simulink model "Quat"  (R2013b)
settings: Solver=ode45  StartTime=0.0  StopTime=100  RelTol=1e-3
undefined symbols (not defined in the file): IMU_DT, MagMeasure, P_init, Q, Rmag, wb, x_init
libraries: simulink x1
settings Model: Creator=Walker  LastModifiedBy=Walker

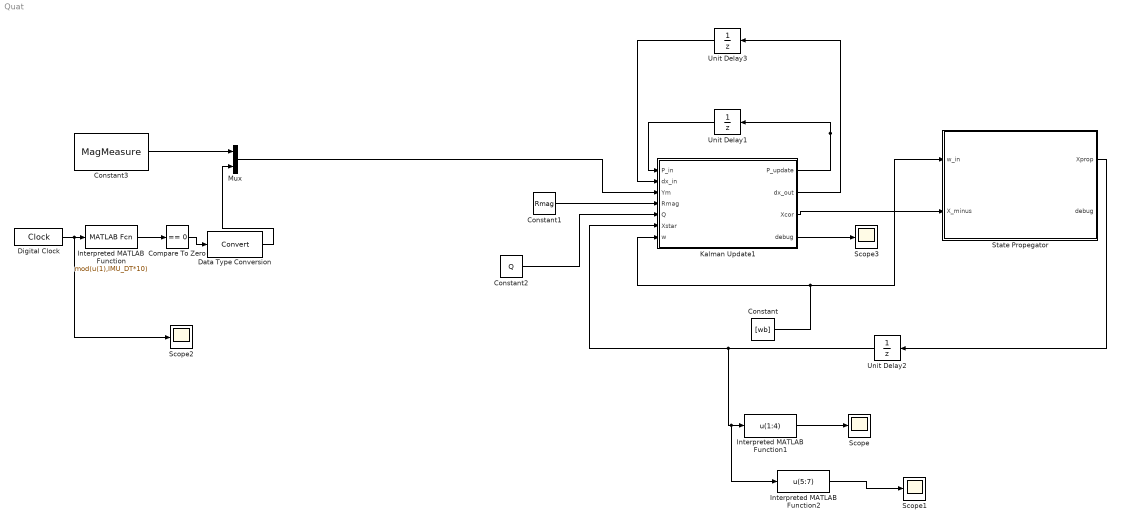
== system Quat ==
  Compare To Zero : simulink/Logic and Bit Operations/Compare To Zero  relop===  OutDataTypeStr=uint8
  Constant : Constant  Value=[wb]
  Constant1 : Constant  Value=Rmag
  Constant2 : Constant  Value=Q
  Constant3 : Constant  Value=MagMeasure
  Data Type Conversion : DataTypeConversion
  Digital Clock : DigitalClock  SampleTime=IMU_DT
  Interpreted MATLAB Function : MATLABFcn  MATLABFcn=mod(u(1),IMU_DT*10)
  Interpreted MATLAB Function1 : MATLABFcn  MATLABFcn=u(1:4)
  Interpreted MATLAB Function2 : MATLABFcn  MATLABFcn=u(5:7)
  Kalman Update1 : MATLAB Function  TreatAsAtomicUnit=on
  Mux : Mux  Inputs=2
  Scope{,1..3} (4 alike) : Scope
      Scope settings: TimeRange=10  YMin=-0.05  YMax=1
      Scope1 settings: YMin=-0.00325  YMax=0.00225
      Scope2 settings: YMin=10  YMax=130  SaveName=ScopeData2
      Scope3 settings: TimeRange=10  YMin=1  YMax=1  SaveName=ScopeData3
  State Propegator : MATLAB Function  TreatAsAtomicUnit=on
  Unit Delay1 : UnitDelay  InitialCondition=P_init  SampleTime=IMU_DT
  Unit Delay2 : UnitDelay  InitialCondition=x_init  SampleTime=IMU_DT
  Unit Delay3 : UnitDelay  InitialCondition=zeros(1,6)  SampleTime=IMU_DT
  wires:
  Kalman Update1/3(Xcor) -> State Propegator/2(X_minus)
  Kalman Update1/1(P_update) -> Unit Delay1/1
  Unit Delay1/1 -> Kalman Update1/1(P_in)
  Constant1/1 -> Kalman Update1/4(Rmag)
  Constant2/1 -> Kalman Update1/5(Q)
  State Propegator/1(Xprop) -> Unit Delay2/1
  Unit Delay2/1 -> Interpreted MATLAB Function2/1, Interpreted MATLAB Function1/1, Kalman Update1/6(Xstar)
  Constant/1 -> State Propegator/1(w_in), Kalman Update1/7(w)
  Constant3/1 -> Mux/1
  Mux/1 -> Kalman Update1/3(Ym)
  Digital Clock/1 -> Scope2/1, Interpreted MATLAB Function/1
  Interpreted MATLAB Function/1 -> Compare To Zero/1
  Unit Delay3/1 -> Kalman Update1/2(dx_in)
  Kalman Update1/2(dx_out) -> Unit Delay3/1
  Compare To Zero/1 -> Data Type Conversion/1
  Data Type Conversion/1 -> Mux/2
  Interpreted MATLAB Function1/1 -> Scope/1
  Interpreted MATLAB Function2/1 -> Scope1/1
  Kalman Update1/4(debug) -> Scope3/1

== matlab function Quat/State Propegator ==
  data: w_in input; X_minus input; Xprop output; debug output
function [   Xprop ,debug ] = TimeUpdate(  w_in  , X_minus) 

   
dt = 1/100;
M = 100;

dt_up = dt/M;



w_b = X_minus(5:7);
qk = X_minus(1:4);

% Apply Correction
w_corr = w_in - w_b;
w1 = w_corr(1);w2 = w_corr(2);w3 = w_corr(3);


for k = 1:M
   q1 = qk(1); q2 = qk(2); q3 = qk(3); q4 = qk(4); 

  
   
   DCM_l2b = [ 1-2*q2*q2-2*q3*q3 , 2*(q1*q2 + q3*q4) , 2*(q3*q1 - q2*q4) ;... 
               2*(q1*q2 - q3*q4) , 1 - 2*q1*q1 - 2*q3*q3 , 2*(q3*q2 + q1*q4) ;...  
               2*(q1*q3 + q2*q4) , 2*(q3*q2 - q1*q4) , 1 - 2*q2*q2 - 2*q1*q1];
   OM = [0 w3 -w2 w1 ; -w3 0 w1 w2 ; w2 -w1 0 w3 ; -w1 -w2 -w3 0 ];
   
  
 
   qdot = .5*OM*qk;
   qk = qdot*dt_up + qk ;
   qk =qk./sqrt(dot(qk,qk));
  
   
end
   
 Xprop = [  qk  ; w_b ];

debug = 0;

== matlab function Quat/Kalman Update1 ==
  data: P_in input; P_update output; dx_in input; dx_out output; Xcor output; debug output; Ym input; Rmag input; Q input; Xstar input; w input
function [ P_update  , dx_out , Xcor, debug] = KamanUpQ(P_in,  dx_in  , Ym  ,Rmag, Q ,   Xstar , w  ) 
coder.extrinsic('.\EKF\linearizeEOM');
coder.extrinsic('.\EKF\PredictMeasurement');
coder.extrinsic('.\EKF\PredictMag');
     

new_mag = Ym(7);
y_mtilde = [0;0;0;0;0;0];
dt = 1/100;
dx_up  = zeros(6,1);

Y_mm = zeros(6,1);


%% Propegate

[A G ] = linearizeEOM( Xstar ,w  );
STM = eye(6) + A*dt;
dx_prop = dx_in;
%dx_prop(7:9) = angErrProp;


P_prop  = STM*P_in*STM' + G*Q*G';
corrApplied = 0;
%% Handle Updates

if new_mag == 1
     Ymag = Ym(1:6);
     [Y_mm Cm DCM1] = predictMag( Xstar );
     Sm = Cm*P_prop*Cm' + Rmag;
     Km = P_prop*Cm'/Sm;
     P_update = P_prop - Km*Cm*P_prop ;
     y_mtilde= Ymag - ( Y_mm  ); 
     dx_up = Km*y_mtilde;
  
     corrApplied = 1;
else
     P_update = P_prop;
end


if corrApplied==1
    
     bias_cor = Xstar(5:7) + dx_up(4:6);
     dAngs =  dx_up(1:3) ;
     quatUp = updateQuat( Xstar(1:4) , dAngs);
    
     Xcor =[   quatUp ; bias_cor  ];
     dx_out = dx_prop + dx_up;     
  
else
    dx_out =dx_prop;
    P_update = P_prop;
    Xcor = Xstar;
end


debug =[dot(Xcor(1:4),Xcor(1:4))];
